simulink model "BDA"  (R2023b)
settings: Solver=VariableStepAuto  StartTime=0.0  StopTime=20  RelTol=1e-3
values from neighbouring files (symbols this model uses):
  G1_den = [1 2]    [BDA_TF.m]    (also in matlab.mat)
  G1_num = [1 0]    [BDA_TF.m]    (also in matlab.mat)
  G2_den = [1 -1]    [BDA_TF.m]    (also in matlab.mat)
  G2_num = [3 6]    [BDA_TF.m]    (also in matlab.mat)
  H_den = [1 -2]    [BDA_TF.m]    (also in matlab.mat)
  H_num = [1 2]    [BDA_TF.m]    (also in matlab.mat)
  TF_den = conv(G_den,G_den_sum)    [BDA_TF.m]    (also in matlab.mat = [4 15 11 -10 -12 -8])
  TF_num = conv(G_num,GH_den)    [BDA_TF.m]    (also in matlab.mat = [3 3 -18 -12 24 0])
settings Model: Creator=Lenovo  LastModifiedBy=Lenovo

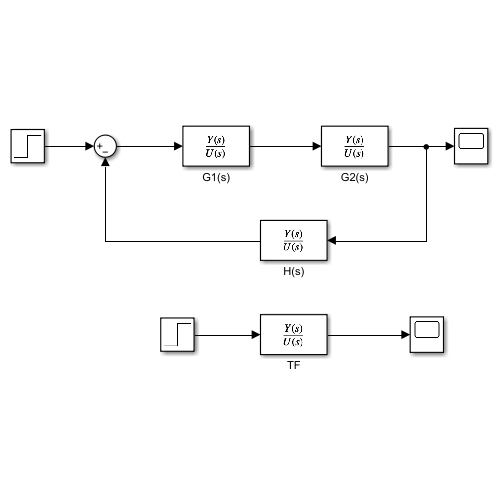
[thumbnail: Simulink's stored preview of the top-level diagram]
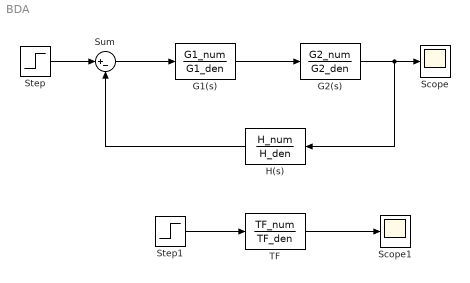
== system BDA ==
  G1(s) : TransferFcn  Numerator=G1_num  Denominator=G1_den
  G2(s) : TransferFcn  Numerator=G2_num  Denominator=G2_den
  H(s) : TransferFcn  Numerator=H_num  Denominator=H_den
  Scope : Scope
  Scope1 : Scope
  Step : Step  Time=0  SampleTime=0
  Step1 : Step  Time=0  SampleTime=0
  Sum : Sum  Inputs=|+-
  TF : TransferFcn  Numerator=TF_num  Denominator=TF_den
  wires:
  Step/1 -> Sum/1
  Sum/1 -> G1(s)/1
  G1(s)/1 -> G2(s)/1
  G2(s)/1 -> H(s)/1, Scope/1
  H(s)/1 -> Sum/2
  Step1/1 -> TF/1
  TF/1 -> Scope1/1
